simulink model "firq_sim_xbits"  (R2019b)
settings: Solver=VariableStepAuto  StartTime=0.0  StopTime=Tstop  RelTol=1e-3
values from neighbouring files (symbols this model uses):
  amp = 0.999    [FIRq_xbitsSNR_sim.m]
  f0 = sigbin*(Fs/N)    (= 437.5)    [FIRq_xbitsSNR_sim.m]
  fir_numq = fir_numq    [FIRq_xbitsSNR_sim.m]
  Ts = 1/Fs    (= 0.000125)    [FIRq_xbitsSNR_sim.m]
settings Model: Creator=straeuss  LastModifiedBy=straeuss
settings DataIOCC: ReturnWorkspaceOutputs=off
settings DebuggingCC: ArithmeticOperatorsInVariantConditions=warning
settings SFSimCC: CustomCodeUndefinedFunction=UseInterfaceOnly

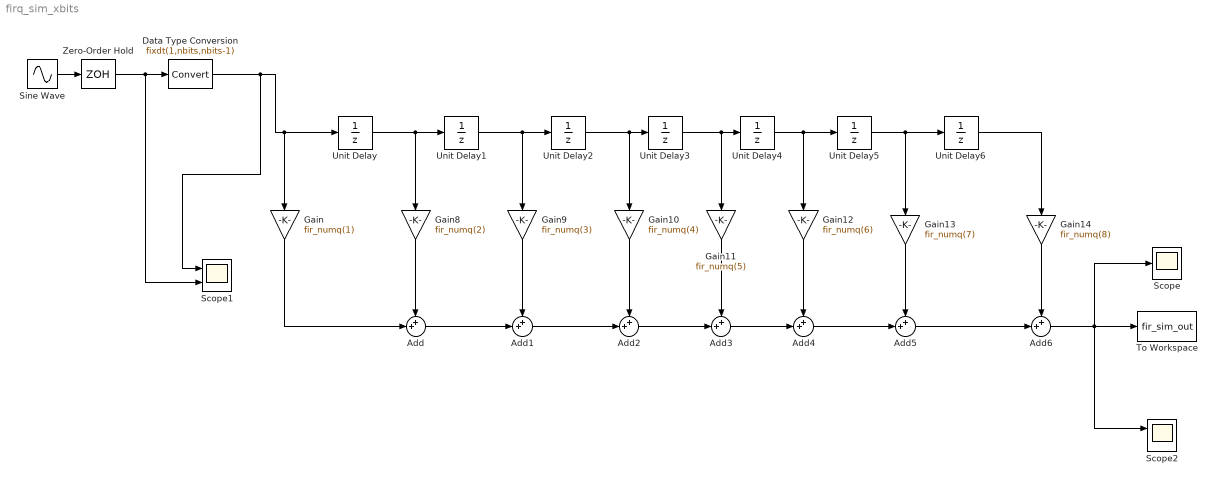
== system firq_sim_xbits ==
  Add{,1..6} (7 alike) : Sum  Inputs=++|  OutDataTypeStr=fixdt(1,nbits_add,nbits+xbits-1)
  Data Type Conversion : DataTypeConversion  OutDataTypeStr=fixdt(1,nbits,nbits-1)
  Gain : Gain  Gain=fir_numq(1)  ParamDataTypeStr=fixdt(1,nbits_coef,nbits_coef-1)  OutDataTypeStr=fixdt(1,nbits+xbits,nbits+xbits-1)
  Gain10 : Gain  Gain=fir_numq(4)  ParamDataTypeStr=fixdt(1,nbits_coef,nbits_coef-1)  OutDataTypeStr=fixdt(1,nbits+xbits,nbits+xbits-1)
  Gain11 : Gain  Gain=fir_numq(5)  ParamDataTypeStr=fixdt(1,nbits_coef,nbits_coef-1)  OutDataTypeStr=fixdt(1,nbits+xbits,nbits+xbits-1)
  Gain12 : Gain  Gain=fir_numq(6)  ParamDataTypeStr=fixdt(1,nbits_coef,nbits_coef-1)  OutDataTypeStr=fixdt(1,nbits+xbits,nbits+xbits-1)
  Gain13 : Gain  Gain=fir_numq(7)  ParamDataTypeStr=fixdt(1,nbits_coef,nbits_coef-1)  OutDataTypeStr=fixdt(1,nbits+xbits,nbits+xbits-1)
  Gain14 : Gain  Gain=fir_numq(8)  ParamDataTypeStr=fixdt(1,nbits_coef,nbits_coef-1)  OutDataTypeStr=fixdt(1,nbits+xbits,nbits+xbits-1)
  Gain8 : Gain  Gain=fir_numq(2)  ParamDataTypeStr=fixdt(1,nbits_coef,nbits_coef-1)  OutDataTypeStr=fixdt(1,nbits+xbits,nbits+xbits-1)
  Gain9 : Gain  Gain=fir_numq(3)  ParamDataTypeStr=fixdt(1,nbits_coef,nbits_coef-1)  OutDataTypeStr=fixdt(1,nbits+xbits,nbits+xbits-1)
  Scope : Scope
  Scope1 : Scope  NumInputPorts=2
  Scope2 : Scope  NumInputPorts=2
  Sine Wave : Sin  Amplitude=amp  Frequency=f0*2*pi  SampleTime=0
  To Workspace : ToWorkspace  VariableName=fir_sim_out  SampleTime=Ts
  Unit Delay{,1..6} (7 alike) : UnitDelay  SampleTime=-1  HasFrameUpgradeWarning=on
  Zero-Order Hold : ZeroOrderHold  SampleTime=-1
  wires:
  Unit Delay/1 -> Gain8/1, Unit Delay1/1
  Unit Delay1/1 -> Unit Delay2/1, Gain9/1
  Unit Delay2/1 -> Gain10/1, Unit Delay3/1
  Unit Delay3/1 -> Unit Delay4/1, Gain11/1
  Unit Delay4/1 -> Gain12/1, Unit Delay5/1
  Unit Delay5/1 -> Gain13/1, Unit Delay6/1
  Gain/1 -> Add/2
  Gain8/1 -> Add/1
  Gain9/1 -> Add1/1
  Gain10/1 -> Add2/1
  Gain11/1 -> Add3/1
  Gain12/1 -> Add4/1
  Gain13/1 -> Add5/1
  Gain14/1 -> Add6/1
  Add/1 -> Add1/2
  Add1/1 -> Add2/2
  Add2/1 -> Add3/2
  Add3/1 -> Add4/2
  Add4/1 -> Add5/2
  Add5/1 -> Add6/2
  Unit Delay6/1 -> Gain14/1
  Add6/1 -> To Workspace/1, Scope/1, Scope2/1
  Zero-Order Hold/1 -> Scope1/2, Data Type Conversion/1
  Data Type Conversion/1 -> Scope1/1, Gain/1, Unit Delay/1
  Sine Wave/1 -> Zero-Order Hold/1
